simulink model "Mondmission"  (R2017b)
settings: Solver=VariableStepAuto  StartTime=0.0  StopTime=864000  RelTol=1e-3
settings Model: Creator=aby032  LastModifiedBy=aby032

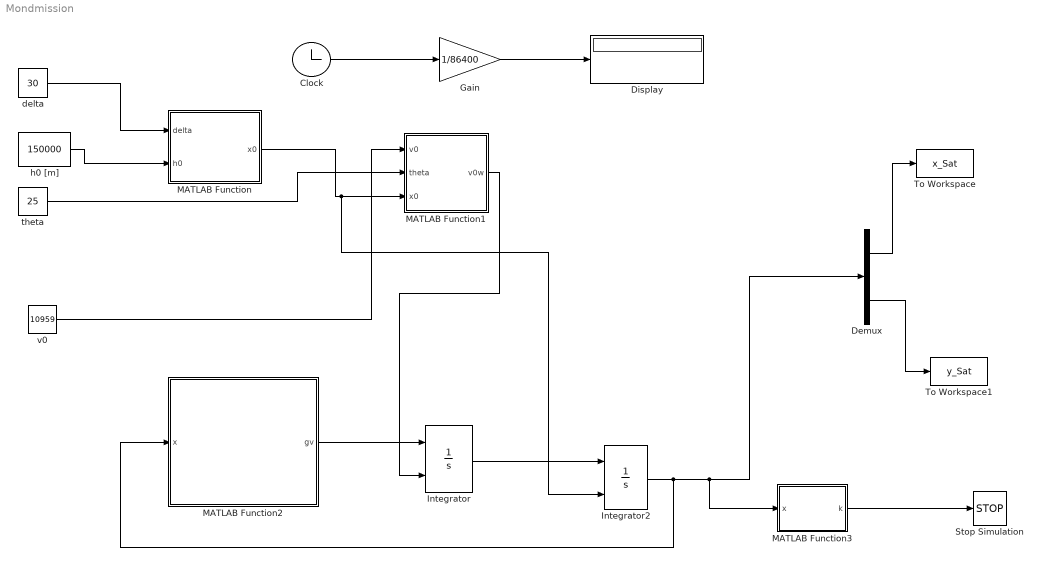
== system Mondmission ==
  Clock : Clock
      settings: Decimation=2
  Demux : Demux  Outputs=2
  Display : Display
  Gain : Gain  Gain=1/86400
  Integrator : Integrator  InitialConditionSource=external
  Integrator2 : Integrator  InitialConditionSource=external
  MATLAB Function : MATLAB Function  TreatAsAtomicUnit=on
  MATLAB Function1 : MATLAB Function  TreatAsAtomicUnit=on
  MATLAB Function2 : MATLAB Function  TreatAsAtomicUnit=on
  MATLAB Function3 : MATLAB Function  TreatAsAtomicUnit=on
  Stop Simulation : Stop
  To Workspace : ToWorkspace  VariableName=x_Sat  SampleTime=-1
      settings: Save2DSignal=2-D array (concatenate along first dimension)
  To Workspace1 : ToWorkspace  VariableName=y_Sat  SampleTime=-1
      settings: Save2DSignal=2-D array (concatenate along first dimension)
  delta : Constant  Value=30
  h0 [m] : Constant  Value=150000
  theta : Constant  Value=25
  v0 : Constant  Value=10959
  wires:
  Clock/1 -> Gain/1
  Gain/1 -> Display/1
  delta/1 -> MATLAB Function/1(delta)
  h0 [m]/1 -> MATLAB Function/2(h0)
  MATLAB Function/1(x0) -> Integrator2/2, MATLAB Function1/3(x0)
  theta/1 -> MATLAB Function1/2(theta)
  v0/1 -> MATLAB Function1/1(v0)
  MATLAB Function1/1(v0w) -> Integrator/2
  MATLAB Function3/1(k) -> Stop Simulation/1
  Demux/1 -> To Workspace/1
  Demux/2 -> To Workspace1/1
  MATLAB Function2/1(gv) -> Integrator/1
  Integrator/1 -> Integrator2/1
  Integrator2/1 -> MATLAB Function2/1(x), MATLAB Function3/1(x), Demux/1

== matlab function Mondmission/MATLAB Function1 ==
  data: v0 input; v0w output; theta input; x0 input
function v0w = vStart(v0,theta,x0)
n = x0/norm(x0);
t = [n(2); -n(1)];

vt = cosd(theta)*v0;
vn = sind(theta)*v0;

v0w = vn*n+vt*t;
end

== matlab function Mondmission/MATLAB Function ==
  data: delta input; x0 output; h0 input
function x0 = Startposition(delta,h0)
re = 6378000; % Erdradius in m

x1 = cosd(delta)*(h0+re)
x2 = sind(delta)*(h0+re)

x0 = [x1; x2]
end

== matlab function Mondmission/MATLAB Function2 ==
  data: x input; gv output
function gv = Gravitation(x)
G = 66.743e-12      % Gravitationskonstante

me = 5.9736e24      % Masse Erde in kg
mm = 7.3480e22      % Masse Mond in kg

p = [0; -380000000]  % Positionsvektor Ende - Mond in m

xb = norm(x);       % Abstand Erde - Satellit in m
xbm = norm(p-x);    % Abstand Satellit - Mond in m

e = x/(-norm(x));   % Einheitsvektor Richtung Satellit -> Erde
em = (p-x)/xbm;     % Einheitvektor Richtung Satellit -> Mond

gve = G*me/(xb*xb)*e
gvm = G*mm/(xbm*xbm)*em
gv = gve+gvm
end

== matlab function Mondmission/MATLAB Function3 ==
  data: x input; k output
function k = Kontakt(x)
re = 6378000
if re < norm(x)
    k = 0
else
    k = 1
end
